simulink model "BLDCTest"  (R2014b)
settings: Solver=ode45  StartTime=0.0  StopTime=3  MaxStep=.001  RelTol=1e-3
values from neighbouring files (symbols this model uses):
  A = A_1 + A_2*currVel(3)    [RobotLqr.m]    (also in RobotLqt.m; motorParams.m = [-r/l,0,0,0)
  B = obj.B    [RobotParams.m]    (also in derive.m = simplify(B); motorParams.m = [2/(3*l),1/(3*l),0)
  C = eye(3)    [RobotLqr.m]    (also in RobotLqt.m; motorParams.m = [1,0,0,0)
  c0 = .001    (= 0.001)    [motorParams.m]
  D = zeros(3, 4)    [RobotLqr.m]    (also in RobotLqt.m; motorParams.m = [0,0,0)
  ke = 1/(285*2*pi/60)    (= 0.0335063038088)    [motorParams.m]
  kt = 33.5e-3    (= 0.0335)    [motorParams.m]
  p = 16    [motorParams.m]
undefined symbols (not defined in the file or in its folder): Vupper
libraries: simulink x1

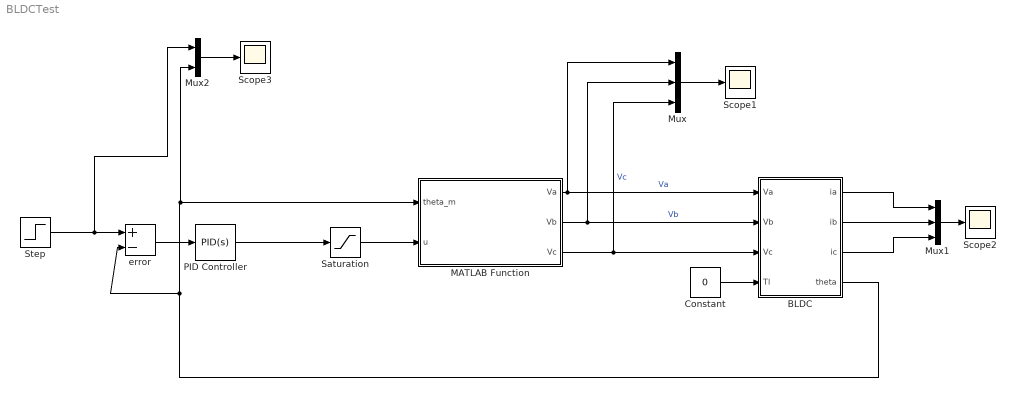
== system BLDCTest ==
  BLDC : Subsystem
  Constant : Constant  Value=0
  MATLAB Function : MATLAB Function  TreatAsAtomicUnit=on
  Mux : Mux  Inputs=3
  Mux1 : Mux  Inputs=3
  Mux2 : Mux  Inputs=2
  PID Controller : simulink/Continuous/PID Controller  Controller=PID  TimeDomain=Continuous-time  SampleTime=-1  IntegratorMethod=Forward Euler  FilterMethod=Forward Euler  Form=Parallel  P=50  I=10  D=0  N=100  InitialConditionSource=internal  InitialConditionForIntegrator=0  InitialConditionForFilter=0  ExternalReset=none  LimitOutput=off  UpperSaturationLimit=inf  LowerSaturationLimit=-inf  LinearizeAsGain=on  AntiWindupMode=none  Kb=1  TrackingMode=off  Kt=1  PParamMin=[]  PParamMax=[]  IParamMin=[]  IParamMax=[]  DParamMin=[]  DParamMax=[]  NParamMin=[]  NParamMax=[]  KbParamMin=[]  KbParamMax=[]  KtParamMin=[]  KtParamMax=[]  POutMin=[]  POutMax=[]  IOutMin=[]  IOutMax=[]  DOutMin=[]  DOutMax=[]  NOutMin=[]  NOutMax=[]  KbOutMin=[]  KbOutMax=[]  KtOutMin=[]  KtOutMax=[]  IntegratorOutMin=[]  IntegratorOutMax=[]  FilterOutMin=[]  FilterOutMax=[]  SumOutMin=[]  SumOutMax=[]  SumI1OutMin=[]  SumI1OutMax=[]  SumI2OutMin=[]  SumI2OutMax=[]  SumI3OutMin=[]  SumI3OutMax=[]  SumDOutMin=[]  SumDOutMax=[]  SaturationOutMin=[]  SaturationOutMax=[]  IntegratorContinuousStateAttributes=''  IntegratorStateMustResolveToSignalObject=off  IntegratorRTWStateStorageClass=Auto  FilterContinuousStateAttributes=''  FilterStateMustResolveToSignalObject=off  FilterRTWStateStorageClass=Auto  DifferentiatorICPrevScaledInput=0  DifferentiatorOutMin=[]  DifferentiatorOutMax=[]  UseFilter=on
  Saturation : Saturate  UpperLimit=Vupper/2  LowerLimit=-Vupper/2
  Scope1 : Scope
  Scope2 : Scope
  Scope3 : Scope
  Step : Step  After=2*pi  SampleTime=0
  error : Sum  Inputs=+-
  wires:
  BLDC/1(ia) -> Mux1/1
  BLDC/2(ib) -> Mux1/2
  BLDC/3(ic) -> Mux1/3
  Constant/1 -> BLDC/4(Tl)
  BLDC/4(theta) -> error/2, Mux2/2, MATLAB Function/1(theta_m)
  Mux1/1 -> Scope2/1
  MATLAB Function/1(Va) -> Mux/1, BLDC/1(Va)  "Va"
  MATLAB Function/2(Vb) -> Mux/2, BLDC/2(Vb)  "Vb"
  MATLAB Function/3(Vc) -> Mux/3, BLDC/3(Vc)  "Vc"
  Mux/1 -> Scope1/1
  error/1 -> PID Controller/1
  Mux2/1 -> Scope3/1
  PID Controller/1 -> Saturation/1
  Saturation/1 -> MATLAB Function/2(u)
  Step/1 -> Mux2/1, error/1

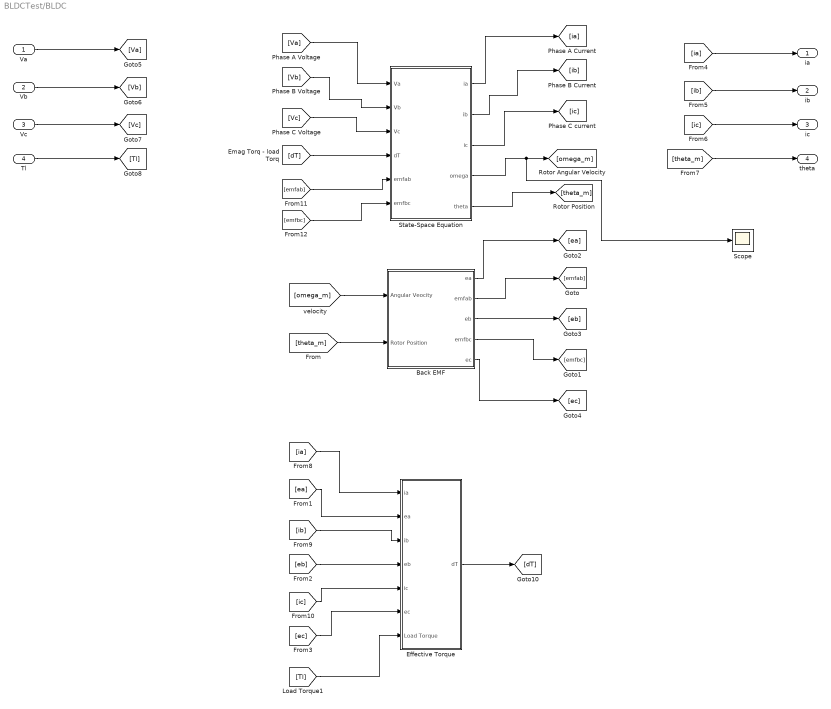
== system BLDCTest/BLDC ==
  Va : Inport
  Vb : Inport  Port=2
  Vc : Inport  Port=3
  Tl : Inport  Port=4
  Back EMF : Subsystem
  Effective Torque : Subsystem
  Scope : Scope
  State-Space Equation : Subsystem
  ia : Outport
  ib : Outport  Port=2
  ic : Outport  Port=3
  theta : Outport  Port=4
  wires:
  State-Space Equation/1(ia) -> [ia]
  [Va] -> State-Space Equation/1(Va)
  State-Space Equation/5(theta) -> [theta_m]
  State-Space Equation/2(ib) -> [ib]
  [dT] -> State-Space Equation/4(dT)
  [Vb] -> State-Space Equation/2(Vb)
  State-Space Equation/4(omega) -> Scope/1, [omega_m]
  State-Space Equation/3(ic) -> [ic]
  [Vc] -> State-Space Equation/3(Vc)
  Effective Torque/1(dT) -> [dT]
  [ib] -> Effective Torque/3(ib)
  [ec] -> Effective Torque/6(ec)
  [ia] -> Effective Torque/1(ia)
  [ea] -> Effective Torque/2(ea)
  [ic] -> Effective Torque/5(ic)
  [Tl] -> Effective Torque/7(Load Torque)
  [eb] -> Effective Torque/4(eb)
  Back EMF/2(emfab) -> [emfab]
  [omega_m] -> Back EMF/1(Angular Veocity)
  Back EMF/5(ec) -> [ec]
  [ib] -> ib/1
  Vc/1 -> [Vc]
  [ic] -> ic/1
  Back EMF/3(eb) -> [eb]
  [theta_m] -> theta/1
  [ia] -> ia/1
  Tl/1 -> [Tl]
  Back EMF/1(ea) -> [ea]
  [theta_m] -> Back EMF/2(Rotor Position)
  Va/1 -> [Va]
  Vb/1 -> [Vb]
  Back EMF/4(emfbc) -> [emfbc]
  [emfab] -> State-Space Equation/5(emfab)
  [emfbc] -> State-Space Equation/6(emfbc)

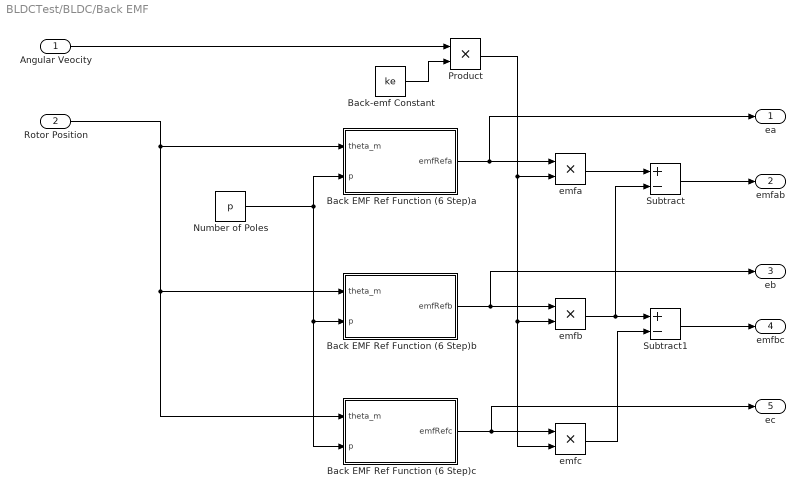
== system BLDCTest/BLDC/Back EMF ==
  Angular Veocity : Inport
  Rotor Position : Inport  Port=2
  Back EMF Ref Function (6 Step)a : MATLAB Function  TreatAsAtomicUnit=on
  Back EMF Ref Function (6 Step)b : MATLAB Function  TreatAsAtomicUnit=on
  Back EMF Ref Function (6 Step)c : MATLAB Function  TreatAsAtomicUnit=on
  Back-emf Constant : Constant  Value=ke
  Number of Poles : Constant  Value=p
  Product : Product
  Subtract : Sum  Inputs=+-
  Subtract1 : Sum  Inputs=+-
  emfa : Product
  emfb : Product
  emfc : Product
  ea : Outport
  emfab : Outport  Port=2
  eb : Outport  Port=3
  emfbc : Outport  Port=4
  ec : Outport  Port=5
  wires:
  Rotor Position/1 -> Back EMF Ref Function (6 Step)a/1(theta_m), Back EMF Ref Function (6 Step)c/1(theta_m), Back EMF Ref Function (6 Step)b/1(theta_m)
  Number of Poles/1 -> Back EMF Ref Function (6 Step)a/2(p), Back EMF Ref Function (6 Step)b/2(p), Back EMF Ref Function (6 Step)c/2(p)
  Back EMF Ref Function (6 Step)a/1(emfRefa) -> ea/1, emfa/1
  emfc/1 -> Subtract1/2
  Back-emf Constant/1 -> Product/2
  Product/1 -> emfa/2, emfc/2, emfb/2
  emfb/1 -> Subtract/2, Subtract1/1
  Back EMF Ref Function (6 Step)b/1(emfRefb) -> eb/1, emfb/1
  Back EMF Ref Function (6 Step)c/1(emfRefc) -> ec/1, emfc/1
  Angular Veocity/1 -> Product/1
  emfa/1 -> Subtract/1
  Subtract/1 -> emfab/1
  Subtract1/1 -> emfbc/1

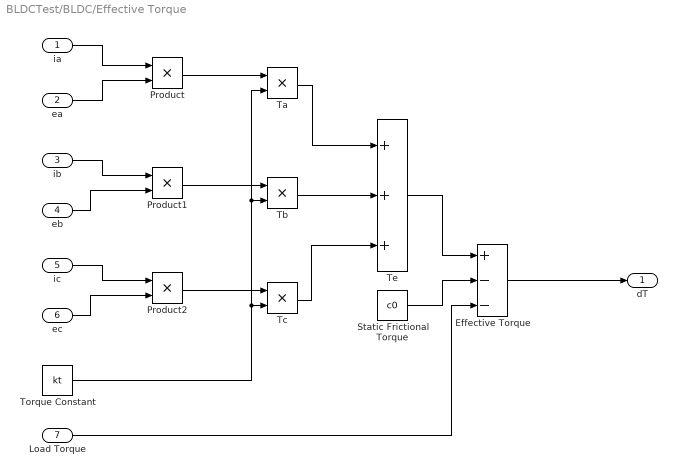
== system BLDCTest/BLDC/Effective Torque ==
  ia : Inport
  ea : Inport  Port=2
  ib : Inport  Port=3
  eb : Inport  Port=4
  ic : Inport  Port=5
  ec : Inport  Port=6
  Load Torque : Inport  Port=7
  Effective Torque : Sum  Inputs=+--
  Product : Product
  Product1 : Product
  Product2 : Product
  Static Frictional Torque : Constant  Value=c0
  Ta : Product  Inputs=**
  Tb : Product  Inputs=**
  Tc : Product  Inputs=**
  Te : Sum  Inputs=+++
  Torque Constant : Constant  Value=kt
  dT : Outport
  wires:
  Static Frictional Torque/1 -> Effective Torque/2
  Load Torque/1 -> Effective Torque/3
  Tc/1 -> Te/3
  Ta/1 -> Te/1
  Tb/1 -> Te/2
  ec/1 -> Product2/2
  eb/1 -> Product1/2
  ib/1 -> Product1/1
  ea/1 -> Product/2
  ic/1 -> Product2/1
  ia/1 -> Product/1
  Effective Torque/1 -> dT/1
  Torque Constant/1 -> Tc/2, Tb/2, Ta/2
  Product/1 -> Ta/1
  Product1/1 -> Tb/1
  Product2/1 -> Tc/1
  Te/1 -> Effective Torque/1

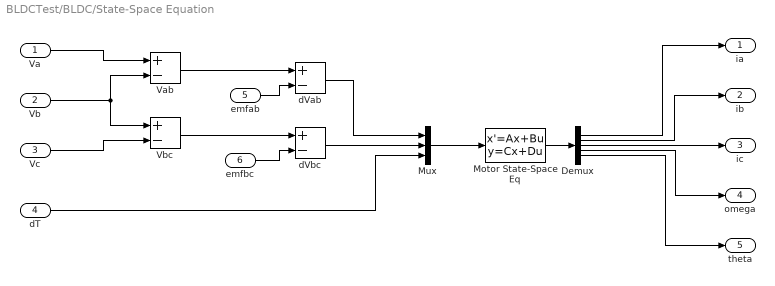
== system BLDCTest/BLDC/State-Space Equation ==
  Va : Inport
  Vb : Inport  Port=2
  Vc : Inport  Port=3
  dT : Inport  Port=4
  emfab : Inport  Port=5
  emfbc : Inport  Port=6
  Demux : Demux  Outputs=5
  Motor State-Space Eq : StateSpace  A=A  B=B  C=C  D=D  X0=0
  Mux : Mux  Inputs=3
  Vab : Sum  Inputs=+-
  Vbc : Sum  Inputs=+-
  dVab : Sum  Inputs=+-
  dVbc : Sum  Inputs=+-
  ia : Outport
  ib : Outport  Port=2
  ic : Outport  Port=3
  omega : Outport  Port=4
  theta : Outport  Port=5
  wires:
  dVbc/1 -> Mux/2
  Demux/2 -> ib/1
  Demux/5 -> theta/1
  Demux/3 -> ic/1
  Demux/1 -> ia/1
  Demux/4 -> omega/1
  Motor State-Space Eq/1 -> Demux/1
  emfbc/1 -> dVbc/2
  Mux/1 -> Motor State-Space Eq/1
  dT/1 -> Mux/3
  Vbc/1 -> dVbc/1
  Vab/1 -> dVab/1
  dVab/1 -> Mux/1
  emfab/1 -> dVab/2
  Va/1 -> Vab/1
  Vb/1 -> Vab/2, Vbc/1
  Vc/1 -> Vbc/2

== matlab function BLDCTest/BLDC/Back EMF/Back EMF Ref Function (6 Step)b ==
function emfRefb = F(theta_m, p)
    theta_e = (p/2).*theta_m - 2*pi/3;
    theta_e = mod(theta_e, (2*pi));
    if theta_e < 0
        theta_e = 2*pi - theta_e;
    end
    if (theta_e <= 2*pi/3)
        emfRefb = 1;
    elseif (theta_e <= pi)
        emfRefb = 1-(6/pi)*(theta_e - 2*pi/3);
    elseif (theta_e <= 5*pi/3)
        emfRefb = -1;
    else
        emfRefb = -1 + (6/pi)*(theta_e - 5*pi/3);
    end

end

== matlab function BLDCTest/BLDC/Back EMF/Back EMF Ref Function (6 Step)a ==
function emfRefa = F(theta_m, p)
    theta_e = (p/2).*theta_m;
    theta_e = mod(theta_e, (2*pi));
    if theta_e < 0
        theta_e = 2*pi - theta_e;
    end
    if (theta_e <= 2*pi/3)
        emfRefa = 1;
    elseif (theta_e <= pi)
        emfRefa = 1-(6/pi)*(theta_e - 2*pi/3);
    elseif (theta_e <= 5*pi/3)
        emfRefa = -1;
    else
        emfRefa = -1 + (6/pi)*(theta_e - 5*pi/3);
    end

end

== matlab function BLDCTest/BLDC/Back EMF/Back EMF Ref Function (6 Step)c ==
function emfRefc = F(theta_m, p)
    theta_e = (p/2).*theta_m + 2*pi/3;
    theta_e = mod(theta_e, (2*pi));
    if theta_e < 0
        theta_e = 2*pi - theta_e;
    end
    if (theta_e <= 2*pi/3)
        emfRefc = 1;
    elseif (theta_e <= pi)
        emfRefc = 1-(6/pi)*(theta_e - 2*pi/3);
    elseif (theta_e <= 5*pi/3)
        emfRefc = -1;
    else
        emfRefc = -1 + (6/pi)*(theta_e - 5*pi/3);
    end

end

== matlab function BLDCTest/MATLAB Function ==
function [Va, Vb, Vc] = halfBridge(theta_m, u)
    poles = 16;
    theta_e = (poles/2)*theta_m;
    theta_e = mod(theta_e, 2*pi);

    if theta_e <= pi/3
        Va = u/2;
        Vb = -u/2;
        Vc = 0;
    elseif theta_e <= 2*pi/3
        Va = u/2;
        Vb = 0;
        Vc = -u/2;
    elseif theta_e <= pi
        Va = 0;
        Vb = u/2;
        Vc = -u/2;
    elseif theta_e <= 4*pi/3
        Va = -u/2;
        Vb = u/2;
        Vc = 0;
    elseif theta_e <= 5*pi/3
        Va = -u/2;
        Vb = 0;
        Vc = u/2;
    else
        Va = 0;
        Vb = -u/2;
        Vc = u/2;
    end
end
